simulink model "logical_operators"  (R2021a)
settings: Solver=VariableStepAuto  StartTime=0.0  StopTime=10.0  RelTol=1e-3
settings Model: Creator=DELL  LastModifiedBy=DELL

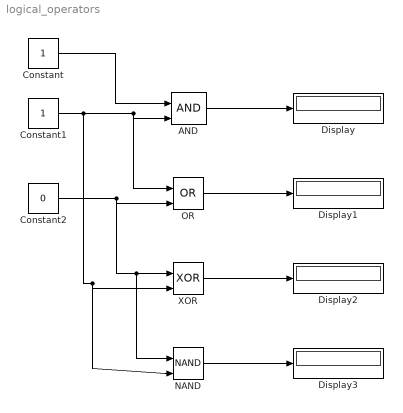
== system logical_operators ==
  AND : Logic  IconShape=distinctive  AllPortsSameDT=off  OutDataTypeStr=boolean
  Constant : Constant
  Constant1 : Constant
  Constant2 : Constant  Value=0
  Display{,1..3} (4 alike) : Display
  NAND : Logic  Operator=NAND  IconShape=distinctive  AllPortsSameDT=off  OutDataTypeStr=boolean
  OR : Logic  Operator=OR  IconShape=distinctive  AllPortsSameDT=off  OutDataTypeStr=boolean
  XOR : Logic  Operator=XOR  IconShape=distinctive  AllPortsSameDT=off  OutDataTypeStr=boolean
  wires:
  Constant1/1 -> NAND/2, XOR/2, OR/1, AND/2
  Constant/1 -> AND/1
  AND/1 -> Display/1
  Constant2/1 -> NAND/1, XOR/1, OR/2
  OR/1 -> Display1/1
  XOR/1 -> Display2/1
  NAND/1 -> Display3/1
